simulink model "m_full_system_model"  (R2022b)
settings: Solver=VariableStepAuto  StartTime=0.0  StopTime=10.0  MaxStep=Tstep  RelTol=1e-3
InitFcn:
  | VDCrated=200;
  | Pbase=10e3;
undefined symbols (not defined in the file): N_r12, N_r13, rfilt
libraries: simulink x4, spspowerguiLib x1
settings Model: Creator=ajunyent  LastModifiedBy=IceSunYX

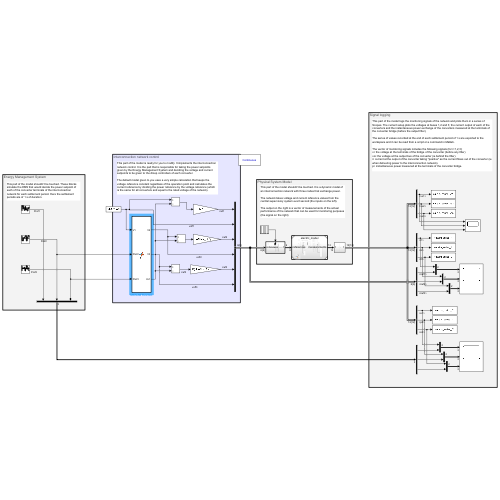
[thumbnail: Simulink's stored preview of the top-level diagram]
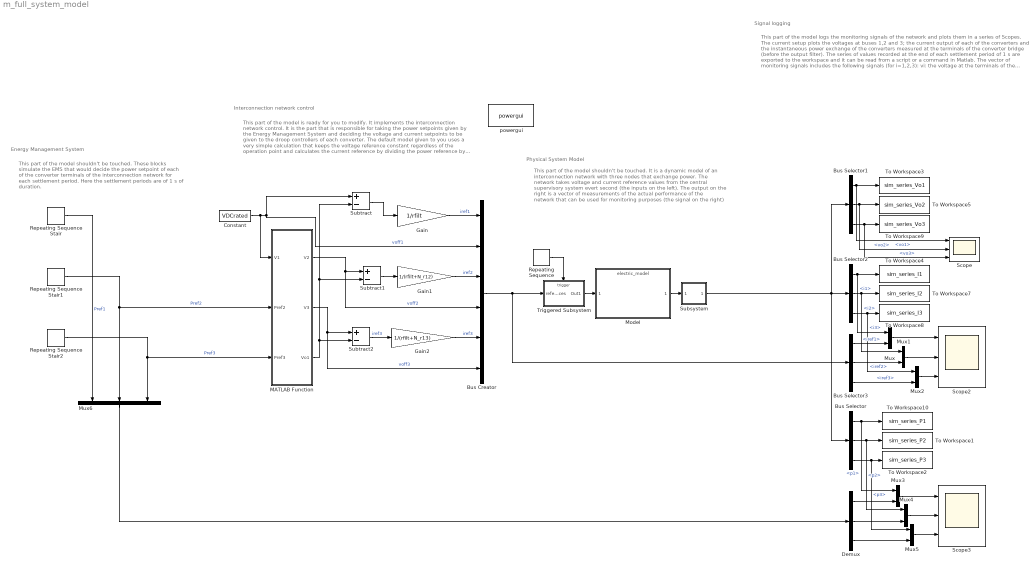
== system m_full_system_model ==
  note: This part of the model is ready for you to modify. It implements the interconnection network control. It is the part that is responsible for taking the power setpoints given by the Energy Management System and deciding the voltage and current setpoints to be given to the droop controllers of each converter.
      |
      | The default model given to you uses a very simple calculation that keeps the voltage reference constant regardless of the operation point and calculates the current reference by dividing the power reference by the voltage reference (which is the same for all converters and equal to the rated voltage of the network).
  note: Interconnection network control
  note: This part of the model shouldn't be touched. These blocks simulate the EMS that would decide the power setpoint of each of the converter terminals of the interconnection network for each settlement period. Here the settlement periods are of 1 s of duration.
  note: Energy Management System
  note: Physical System Model
  note: This part of the model shouldn't be touched. It is a dynamic model of an interconnection network with three nodes that exchange power.
      |
      | The network takes voltage and current reference values from the central supervisory system evert second (the inputs on the left).
      |
      | The output on the right is a vector of measurements of the actual performance of the network that can be used for monitoring purposes (the signal on the right)
  note: This part of the model logs the monitoring signals of the network and plots them in a series of Scopes. The current setup plots the voltages at buses 1,2 and 3; the current output of each of the converters and the instantaneous power exchange of the converters measured at the terminals of the converter bridge (before the output filter).
      |
      | The series of values recorded at the end of each settlement period of 1 s are exported to the workspace and it can be read from a script or a command in Matlab.
      |
      | The vector of monitoring signals includes the following signals (for i=1,2,3):
      | vi: the voltage at the terminals of the bridge of the converter (before any filter)
      | voi: the voltage at the output bus of the converter (ie behind the filter).
      | ii: current at the output of the converter taking "positive" as the current flows out of the converter (ie when delivering power to the interconnection network).
      | pi: instantaneous power measured at the terminals of the converter bridge.
  note: Signal logging
  Bus Creator : BusCreator  Inputs=6
  Bus Selector : BusSelector  OutputSignals=p1,p2,p3
  Bus Selector1 : BusSelector  OutputSignals=vo1,vo2,vo3
  Bus Selector2 : BusSelector  OutputSignals=i1,i2,i3
  Bus Selector3 : BusSelector  OutputSignals=iref1,iref2,iref3
  Constant : Constant  Value=VDCrated
  Demux : Demux  Outputs=3
  Gain : Gain  Gain=1/rfilt
  Gain1 : Gain  Gain=1/(rfilt+N_r12)
  Gain2 : Gain  Gain=1/(rfilt+N_r13)
  MATLAB Function : MATLAB Function  TreatAsAtomicUnit=on
  Model : ModelReference  ModelNameDialog=electric_model.slx  SimulationMode=Normal  ModelReferenceVersion=2.2
  Mux{,1..5} (6 alike) : Mux  Inputs=2
  Mux6 : Mux  Inputs=3
  Repeating Sequence : simulink/Sources/Repeating Sequence  rep_seq_t=[0 0.005 0.006 0.5 0.501 1]  rep_seq_y=[0,0,1 1 0 0]
  Repeating Sequence Stair : simulink/Sources/Repeating Sequence Stair  OutValues=seriesP1ref  tsamp=1  OutMin=[]  OutMax=[]  OutDataTypeStr=double  OutputDataTypeScalingMode=double  OutDataType=fixdt(0,8)  ConRadixGroup=Best Precision: Vector-wise  OutScaling=2^-12
  Repeating Sequence Stair1 : simulink/Sources/Repeating Sequence Stair  OutValues=seriesP2ref  tsamp=1  OutMin=[]  OutMax=[]  OutDataTypeStr=double  OutputDataTypeScalingMode=double  OutDataType=fixdt(0,8)  ConRadixGroup=Best Precision: Vector-wise  OutScaling=2^-12
  Repeating Sequence Stair2 : simulink/Sources/Repeating Sequence Stair  OutValues=seriesP3ref  tsamp=1  OutMin=[]  OutMax=[]  OutDataTypeStr=double  OutputDataTypeScalingMode=double  OutDataType=fixdt(0,8)  ConRadixGroup=Best Precision: Vector-wise  OutScaling=2^-12
  Scope : Scope  NumInputPorts=3
  Scope2 : Scope  NumInputPorts=3
  Scope3 : Scope  NumInputPorts=3
  Subsystem : Subsystem
  Subtract : Sum  Inputs=+-
  Subtract1 : Sum  Inputs=+-
  Subtract2 : Sum  Inputs=+-
  To Workspace1 : ToWorkspace  VariableName=sim_series_P2  SampleTime=1
      settings: MaxDataPoints=10
  To Workspace10 : ToWorkspace  VariableName=sim_series_P1  SampleTime=1
      settings: MaxDataPoints=10
  To Workspace2 : ToWorkspace  VariableName=sim_series_P3  SampleTime=1
      settings: MaxDataPoints=10
  To Workspace3 : ToWorkspace  VariableName=sim_series_Vo1  SampleTime=1
      settings: MaxDataPoints=10
  To Workspace4 : ToWorkspace  VariableName=sim_series_I1  SampleTime=1
      settings: MaxDataPoints=10
  To Workspace5 : ToWorkspace  VariableName=sim_series_Vo2  SampleTime=1
      settings: MaxDataPoints=10
  To Workspace7 : ToWorkspace  VariableName=sim_series_I2  SampleTime=1
      settings: MaxDataPoints=10
  To Workspace8 : ToWorkspace  VariableName=sim_series_I3  SampleTime=1
      settings: MaxDataPoints=10
  To Workspace9 : ToWorkspace  VariableName=sim_series_Vo3  SampleTime=1
      settings: MaxDataPoints=10
  Triggered Subsystem : Subsystem  TreatAsAtomicUnit=on
  powergui : spspowerguiLib/powergui  Priority=1  SimulationMode=Continuous  SampleTime=50e-6  frequency=60  Iterations=50  frequencyindice=0  Pbase=100e6  ErrMax=1e-4  UnitsV=kV  UnitsW=MW  buscounter=0  FunctionMessages=off  echomessages=off  EnableUseOfTLC=off  CurrentSourceSwitches=off  DisableSnubberDevices=off  DisableRonSwitches=off  DisableVfSwitches=off  DisplayEquations=off  AutomaticDiscreteSolvers=off  SolverType=Tustin/Backward Euler (TBE)  Interpol=off  ExternalGateDelay=off  methode=off  Ts=100  x0status=blocks  SPID=on  SwTol=0  HookPort=off  NonlinearTolerance=1e-4  nMaxIteration=100  ContinueOnMaxIteration=off  RestoreLinks=warning  ResistiveCurrentMeasurement=off  Frange=[0:2:500]  Ylog=off  Xlog=on  ShowGrid=off  save=off  variable=ZData  structure=0  ZoomFFT=off  StartTime=0.0  cycles=1  DisplayStyle=1  fundamental=60  FreqAxis=off  MaxFrequency=1000  frequencyindicesteady=1  RmsSteady=1  display=off
  wires:
  Constant/1 -> MATLAB Function/1(V1), Subtract/1, Bus Creator/2  "voff1"
  Repeating Sequence Stair1/1 -> Mux6/2, MATLAB Function/2(Pref2)  "Pref2"
  Gain2/1 -> Bus Creator/5  "iref3"
  MATLAB Function/2(V3) -> Subtract2/1, Bus Creator/6  "voff3"
  Model/1 -> Subsystem/1(In1)
  Triggered Subsystem/1(Out1) -> Model/1
  Repeating Sequence Stair/1 -> Mux6/1  "Pref1"
  Repeating Sequence/1 -> Triggered Subsystem/Trigger
  MATLAB Function/1(V2) -> Subtract1/1, Bus Creator/4  "voff2"
  Bus Selector2/3 -> To Workspace8/1, Mux2/1  "<i3>"
  Bus Creator/1 -> Triggered Subsystem/1(references), Bus Selector3/1
  Bus Selector/1 -> To Workspace10/1, Mux3/1  "<p1>"
  Mux/1 -> Scope2/1
  Bus Selector2/2 -> To Workspace7/1, Mux1/1  "<i2>"
  Subsystem/1(Out1) -> Bus Selector1/1, Bus Selector2/1, Bus Selector/1
  Bus Selector1/3 -> To Workspace9/1, Scope/3  "<vo3>"
  Bus Selector/3 -> To Workspace2/1, Mux5/1  "<p3>"
  Mux2/1 -> Scope2/3
  Bus Selector/2 -> To Workspace1/1, Mux4/1  "<p2>"
  Bus Selector3/2 -> Mux1/2  "<iref2>"
  Bus Selector1/1 -> To Workspace3/1, Scope/1  "<vo1>"
  Bus Selector3/1 -> Mux/2  "<iref1>"
  Bus Selector3/3 -> Mux2/2  "<iref3>"
  Bus Selector1/2 -> To Workspace5/1, Scope/2  "<vo2>"
  Mux1/1 -> Scope2/2
  Bus Selector2/1 -> To Workspace4/1, Mux/1  "<i1>"
  Mux4/1 -> Scope3/2
  Mux5/1 -> Scope3/3
  Mux3/1 -> Scope3/1
  Demux/1 -> Mux3/2
  Demux/2 -> Mux4/2
  Demux/3 -> Mux5/2
  Gain/1 -> Bus Creator/1  "iref1"
  Gain1/1 -> Bus Creator/3  "iref2"
  Repeating Sequence Stair2/1 -> MATLAB Function/3(Pref3), Mux6/3  "Pref3"
  Mux6/1 -> Demux/1
  MATLAB Function/3(Vo1) -> Subtract2/2, Subtract1/2, Subtract/2
  Subtract/1 -> Gain/1
  Subtract1/1 -> Gain1/1
  Subtract2/1 -> Gain2/1  "iref3"

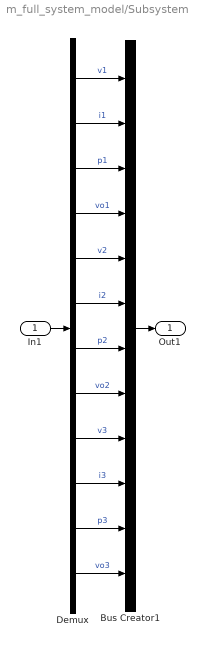
== system m_full_system_model/Subsystem ==
  In1 : Inport
  Bus Creator1 : BusCreator  Inputs=12
  Demux : Demux  Outputs=12
  Out1 : Outport
  wires:
  Demux/2 -> Bus Creator1/2  "i1"
  Bus Creator1/1 -> Out1/1
  Demux/4 -> Bus Creator1/4  "vo1"
  Demux/1 -> Bus Creator1/1  "v1"
  Demux/11 -> Bus Creator1/11  "p3"
  Demux/5 -> Bus Creator1/5  "v2"
  In1/1 -> Demux/1
  Demux/10 -> Bus Creator1/10  "i3"
  Demux/8 -> Bus Creator1/8  "vo2"
  Demux/7 -> Bus Creator1/7  "p2"
  Demux/3 -> Bus Creator1/3  "p1"
  Demux/12 -> Bus Creator1/12  "vo3"
  Demux/9 -> Bus Creator1/9  "v3"
  Demux/6 -> Bus Creator1/6  "i2"

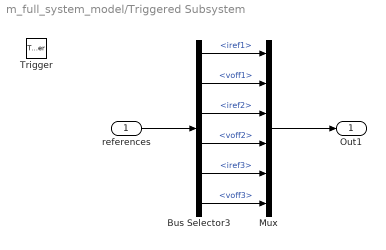
== system m_full_system_model/Triggered Subsystem ==
  references : Inport
  Trigger : TriggerPort  VariantControl=(inherit)  InitialTriggerSignalState=zero
  Bus Selector3 : BusSelector  OutputSignals=iref1,voff1,iref2,voff2,iref3,voff3
  Mux : Mux  Inputs=6
  Out1 : Outport  InitialOutput=[0,VDCrated,0,VDCrated,0,VDCrated]
  wires:
  Bus Selector3/2 -> Mux/2  "<voff1>"
  Bus Selector3/4 -> Mux/4  "<voff2>"
  Bus Selector3/1 -> Mux/1  "<iref1>"
  Bus Selector3/5 -> Mux/5  "<iref3>"
  Bus Selector3/6 -> Mux/6  "<voff3>"
  Mux/1 -> Out1/1
  Bus Selector3/3 -> Mux/3  "<iref2>"
  references/1 -> Bus Selector3/1

== matlab function m_full_system_model/MATLAB Function ==
  data: V1 input; V2 output; Pref2 input; Pref3 input; V3 output; Vo1 output
function [V2,V3,Vo1] = fcn(V1,Pref2,Pref3)
    R_1 = 0.09;
    R_2 = 0.09;
    R_3 = 0.09;
    R_12 = 0.05;
    R_13 = 0.04;
    
    G22 = 1 / (R_12 + R_2);
    G24 = -1 / (R_12 + R_2);
    G33 = 1 / (R_13 + R_3);
    G34 = -1 / (R_13 + R_3);
    G41 = -1 / R_1;
    G42 = -1 / (R_12 + R_2);
    G43 = -1 / (R_13 + R_3);
    G44 = 1 / R_1 + 1 / (R_12 + R_2) + 1 / (R_13 + R_3);
    
    f = @(V2,V3,Vo1) [V2*V2*G22+V2*Vo1*G24-Pref2;
                     V3*V3*G33+V3*Vo1*G34-Pref3;
                     Vo1*V1*G41+Vo1*V2*G42+Vo1*V3*G43+Vo1*Vo1*G44];
                 
    fp = @(x) f(x(1), x(2), x(3));
    options = optimoptions('fsolve', 'Algorithm', 'Levenberg-Marquardt');
    [x, fval] = fsolve(fp, [200; 200; 200], options);
    disp(x);
    
    V2 = x(1);
    V3 = x(2);
    Vo1 = x(3);
end
